simulink model "flightgear"  (R2021a)
settings: Solver=VariableStepAuto  StartTime=0.0  StopTime=10.0  RelTol=1e-3
undefined symbols (not defined in the file): Earth, WGS84
libraries: aerolibfltsims x2, shared6dof x1, aerolibtransform2 x1
settings Model: Creator=muhammed  LastModifiedBy=muhammed

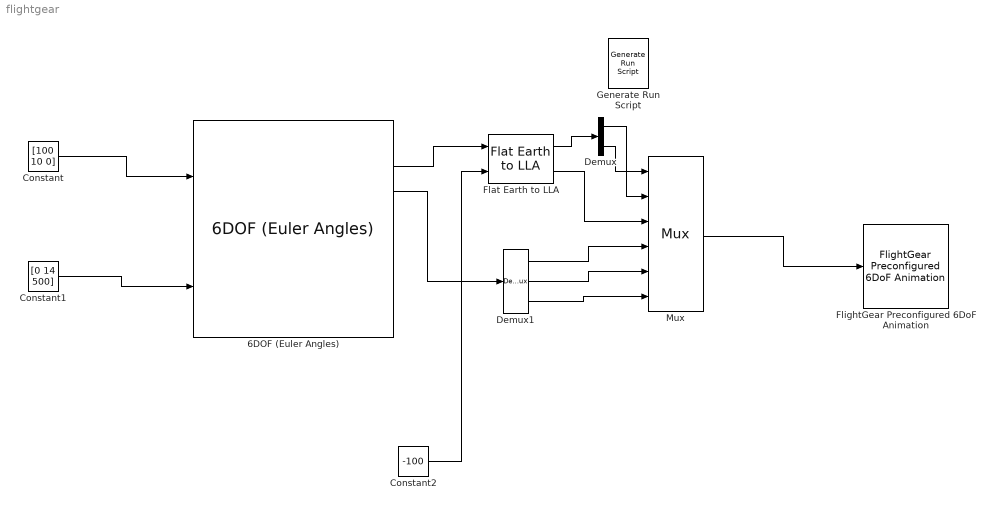
== system flightgear ==
  6DOF (Euler Angles) : shared6dof/6DOF (Euler Angles)  units=Metric (MKS)  mtype=Fixed  rep=Euler Angles  xme_0=[0 0 0]  Vm_0=[0 0 0]  eul_0=[0 0 0]  pm_0=[0 0 0]  mass_0=1.0  mass_e=0.5  mass_f=2.0  inertia=eye(3)  inertia_e=eye(3)  inertia_f=2*eye(3)  k_quat=1.0  vre_flag=on  abi_flag=off  aMode=0  xme_statename=''  Vm_statename=''  eul_statename=''  quat_statename=''  pm_statename=''  mass_statename=''
      settings: SourceProductBaseCode=AE,PW,DR,MT,UV,VE
  Constant : Constant  Value=[100 10 0]
  Constant1 : Constant  Value=[0 14 500]
  Constant2 : Constant  Value=-100
  Demux : Demux  Outputs=2
  Demux1 : Demux  Outputs=3
  Flat Earth to LLA : aerolibtransform2/Flat Earth to LLA  units=Metric (MKS)  ptype=Earth (WGS84)  F=1/298.257223563  R=6378137  refPosPort=off  LL0=[0 10]  psi=0
  FlightGear Preconfigured 6DoF Animation : aerolibfltsims/FlightGear Preconfigured 6DoF Animation  xFlightGearVersion=v2019.1  DestinationIpAddress=127.0.0.1  DestinationPort=5502  SampleTime=1/30  packetVersion=24
  Generate Run Script : aerolibfltsims/Generate Run Script  Architecture=Default  dataFlow=Send  GeometryModelName=c172p  AirportId=KSFO  RunwayId=10L  InitialAltitude=7224  InitialHeading=113  OffsetDistance=4.72  OffsetAzimuth=0  InstallScenery=off  DisableShaders=off  OriginAddress=127.0.0.1  DestinationPort=5502  OriginPort=5505  LocalAddress=127.0.0.1  OutputFileName=runfg1.bash  FlightGearBaseDirectory=/usr/share/games
  Mux : Mux  Inputs=6
  wires:
  Constant/1 -> 6DOF (Euler Angles)/1
  Constant1/1 -> 6DOF (Euler Angles)/2
  Mux/1 -> FlightGear Preconfigured 6DoF Animation/1
  6DOF (Euler Angles)/2 -> Flat Earth to LLA/1
  Constant2/1 -> Flat Earth to LLA/2
  Flat Earth to LLA/1 -> Demux/1
  Demux/1 -> Mux/2
  Demux/2 -> Mux/1
  Flat Earth to LLA/2 -> Mux/3
  6DOF (Euler Angles)/3 -> Demux1/1
  Demux1/1 -> Mux/4
  Demux1/2 -> Mux/5
  Demux1/3 -> Mux/6
